simulink model "reciprocity"  (R2015a)
settings: Solver=ode45  StartTime=0.0  StopTime=10.0  RelTol=1e-3
libraries: fl_lib x12, nesl_utility x4
settings Model: Creator=ASUS  LastModifiedBy=ASUS

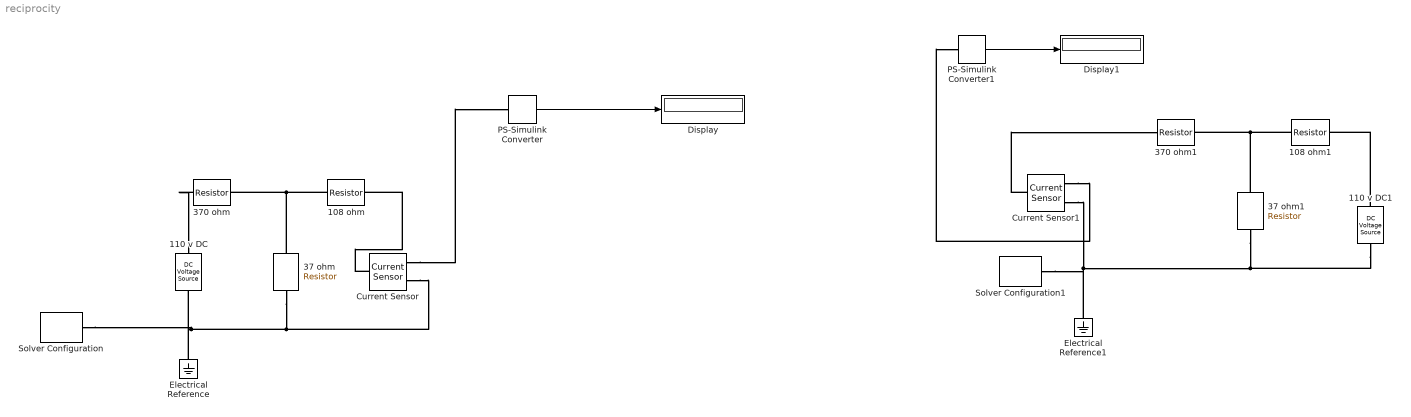
== system reciprocity ==
  " 108 ohm" : fl_lib/Electrical/Electrical Elements/Resistor  R=108 Ohm  i_specify=off  i_priority=High  i=0 A  v_specify=off  v_priority=High  v=0 V
  " 108 ohm1" : fl_lib/Electrical/Electrical Elements/Resistor  R=108 Ohm  i_specify=off  i_priority=High  i=0 A  v_specify=off  v_priority=High  v=0 V
  110 v DC : fl_lib/Electrical/Electrical Sources/DC Voltage Source  v0=110 V
  110 v DC1 : fl_lib/Electrical/Electrical Sources/DC Voltage Source  v0=110 V
  37 ohm : fl_lib/Electrical/Electrical Elements/Resistor  R=37 Ohm  i_specify=off  i_priority=High  i=0 A  v_specify=off  v_priority=High  v=0 V
  37 ohm1 : fl_lib/Electrical/Electrical Elements/Resistor  R=37 Ohm  i_specify=off  i_priority=High  i=0 A  v_specify=off  v_priority=High  v=0 V
  370 ohm : fl_lib/Electrical/Electrical Elements/Resistor  R=370 Ohm  i_specify=off  i_priority=High  i=0 A  v_specify=off  v_priority=High  v=0 V
  370 ohm1 : fl_lib/Electrical/Electrical Elements/Resistor  R=370 Ohm  i_specify=off  i_priority=High  i=0 A  v_specify=off  v_priority=High  v=0 V
  Current Sensor : fl_lib/Electrical/Electrical Sensors/Current Sensor
  Current Sensor1 : fl_lib/Electrical/Electrical Sensors/Current Sensor
  Display : Display
  Display1 : Display
  Electrical Reference : fl_lib/Electrical/Electrical Elements/Electrical Reference
  Electrical Reference1 : fl_lib/Electrical/Electrical Elements/Electrical Reference
  PS-Simulink Converter : nesl_utility/PS-Simulink Converter  PhysicalDomain=network_engine_domain  SubClassName=ps_output  LeftPortType=input  RightPortType=output  PseudoPeriodic=off  Frequencies=[]  Unit=1  AffineConversion=off
  PS-Simulink Converter1 : nesl_utility/PS-Simulink Converter  PhysicalDomain=network_engine_domain  SubClassName=ps_output  LeftPortType=input  RightPortType=output  PseudoPeriodic=off  Frequencies=[]  Unit=1  AffineConversion=off
  Solver Configuration : nesl_utility/Solver Configuration  PhysicalDomain=network_engine_domain  SubClassName=solver  LeftPortType=input  RightPortType=generic  Accelerate=off  Tones=[]  Harmonics=[]  SimulateNoise=off  Profile=off  UseLocalSampling=off  EnableSwitchedLinearOptims=on  FrequencyDomain=off  UseCCode=off  RelTol=0.001  AbsTol=1e-06  MinStep=1e-09  ToWorkspace=off  RevertToSquareIcSolve=off  NumHomotopyIterations=100  DoDC=off  ResidualTolerance=1e-09  UseLocalSolver=off  LocalSolverChoice=NE_BACKWARD_EULER_ADVANCER  LocalSolverSampleTime=0.001  DoFixedCost=off  MaxNonlinIter=3  MaxModeIter=2  LinearAlgebra=Sparse  DelaysMemoryBudget=1024  AutomaticFiltering=on  FilteringTimeConstant=0.001
  Solver Configuration1 : nesl_utility/Solver Configuration  PhysicalDomain=network_engine_domain  SubClassName=solver  LeftPortType=input  RightPortType=generic  Accelerate=off  Tones=[]  Harmonics=[]  SimulateNoise=off  Profile=off  UseLocalSampling=off  EnableSwitchedLinearOptims=on  FrequencyDomain=off  UseCCode=off  RelTol=0.001  AbsTol=1e-06  MinStep=1e-09  ToWorkspace=off  RevertToSquareIcSolve=off  NumHomotopyIterations=100  DoDC=off  ResidualTolerance=1e-09  UseLocalSolver=off  LocalSolverChoice=NE_BACKWARD_EULER_ADVANCER  LocalSolverSampleTime=0.001  DoFixedCost=off  MaxNonlinIter=3  MaxModeIter=2  LinearAlgebra=Sparse  DelaysMemoryBudget=1024  AutomaticFiltering=on  FilteringTimeConstant=0.001
  wires:
  PS-Simulink Converter/1 -> Display/1
  PS-Simulink Converter1/1 -> Display1/1
  connections:
  37 ohm/RConn1 -- Electrical Reference/LConn1 -- 110 v DC/RConn1 -- Solver Configuration/RConn1 -- Current Sensor/RConn2
  370 ohm/LConn1 -- 110 v DC/LConn1
  37 ohm/LConn1 -- " 108 ohm"/LConn1 -- 370 ohm/RConn1
  Current Sensor/RConn1 -- PS-Simulink Converter/LConn1
  Current Sensor/LConn1 -- " 108 ohm"/RConn1
  37 ohm1/RConn1 -- Solver Configuration1/RConn1 -- Electrical Reference1/LConn1 -- Current Sensor1/RConn2 -- 110 v DC1/RConn1
  37 ohm1/LConn1 -- " 108 ohm1"/LConn1 -- 370 ohm1/RConn1
  Current Sensor1/LConn1 -- 370 ohm1/LConn1
  110 v DC1/LConn1 -- " 108 ohm1"/RConn1
  Current Sensor1/RConn1 -- PS-Simulink Converter1/LConn1
